simulink model "model_450"  (R2019b)
settings: Solver=VariableStepAuto  StartTime=0.0  StopTime=10  RelTol=3
libraries: powerlib x15, powerlib_meascontrol x3, eePwmGenerator x1
settings Model: Creator=Администратор  LastModifiedBy=Андрей
settings SFSimCC: CustomCodeUndefinedFunction=UseInterfaceOnly

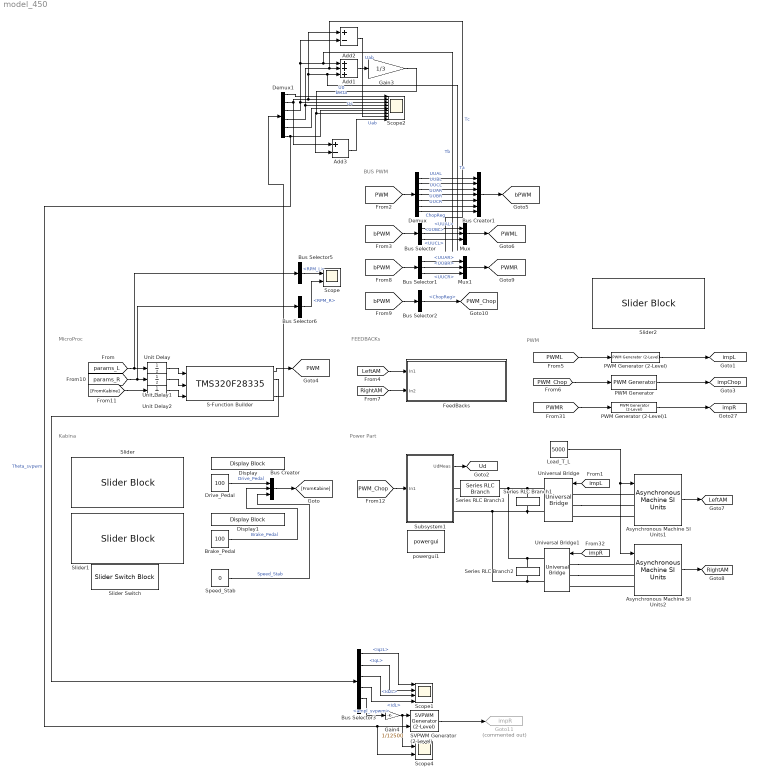
== system model_450 ==
  note: MiсroProc
  note: Kabina
  note: FEEDBACKs
  note: PWM
  note: Power Part
  note: BUS PWM
  Add1 : Sum  Inputs=+++
  Add2 : Sum  Inputs=+-
  Add3 : Sum  Inputs=+-
  Asynchronous Machine SI Units1 : powerlib/Machines/Asynchronous Machine SI Units  RotorType=Squirrel-cage  PresetModel=No  MechanicalLoad=Torque Tm  ShowDetailedParameters=on  ReferenceFrame=Rotor  Units=SI  MeasurementBus=off  NominalParameters=[800000 425 30]  Stator=[0.005 0.00015]  Rotor=[0.00483 0.00015]  Cage1=[ 0.022 0.226/377]  Cage2=[ 0.022 0.226/377]  Lm=0.0072  Mechanical=[100 0 3]  PolePairs=2  InitialConditions=[1 0 0 0 0 0 0 0]  SimulateSaturation=off  Saturation=[14.03593122, 27.81365428, 53.79336849, 72.68890987, 97.98006896, 148.6815601, 215.7428561, 302.9841135, 420.4778367 ; 230, 322, 414, 460, 506, 552, 598, 644, 690]  LoadFlowParameters=1492000  TsPowergui=0  TsBlock=-1  IterativeModel=Trapezoidal non iterative  IterativeDiscreteModel=Trapezoidal non iterative  Pmec=0
      settings: SourceProductName=Simscape Electrical
  Asynchronous Machine SI Units2 : powerlib/Machines/Asynchronous Machine SI Units  RotorType=Squirrel-cage  PresetModel=No  MechanicalLoad=Torque Tm  ShowDetailedParameters=on  ReferenceFrame=Rotor  Units=SI  MeasurementBus=off  NominalParameters=[800000 425 30]  Stator=[0.005 0.00015]  Rotor=[0.00483 0.00015]  Cage1=[ 0.022 0.226/377]  Cage2=[ 0.022 0.226/377]  Lm=0.0072  Mechanical=[100 0 3]  PolePairs=2  InitialConditions=[1 0 0 0 0 0 0 0]  SimulateSaturation=off  Saturation=[14.03593122, 27.81365428, 53.79336849, 72.68890987, 97.98006896, 148.6815601, 215.7428561, 302.9841135, 420.4778367 ; 230, 322, 414, 460, 506, 552, 598, 644, 690]  LoadFlowParameters=1492000  TsPowergui=0  TsBlock=-1  IterativeModel=Trapezoidal non iterative  IterativeDiscreteModel=Trapezoidal non iterative  Pmec=0
      settings: SourceProductName=Simscape Electrical
  Brake_Pedal : Constant  Value=100
  Bus Creator : BusCreator  Inputs=3
  Bus Creator1 : BusCreator  Inputs=7
  Bus Selector : BusSelector  OutputSignals=UUAL,UUBL,UUCL
  Bus Selector1 : BusSelector  OutputSignals=UUAR,UUBR,UUCR
  Bus Selector2 : BusSelector  OutputSignals=ChopReg
  Bus Selector3 : BusSelector  OutputSignals=IqzL,IqL,IdzL,IdL,ampl_svpwm,fThetaL
  Bus Selector5 : BusSelector  OutputSignals=RPM_L
  Bus Selector6 : BusSelector  OutputSignals=RPM_R
  Demux : Demux  Outputs=7
  Demux1 : Demux  Outputs=6
  Display : DisplayBlock  LabelPosition=Hide  Format=short
  Display1 : DisplayBlock  LabelPosition=Hide  Format=short
  Drive_Pedal : Constant  Value=100
  FeedBacks : Subsystem
  Gain3 : Gain  Gain=1/3
  Gain4 : Gain  Gain=1/12500
  Goto11 : Goto  Commented=on  GotoTag=impR  TagVisibility=global
  Load_T_L : Constant  Value=5000
  Mux : Mux  Inputs=3
  Mux1 : Mux  Inputs=3
  PWM Generator : eePwmGenerator/PWM Generator  CarrCount=Up  Tper=0.000666  Ts=1e-5
      settings: SourceProductName=Simscape Electrical
  PWM Generator (2-Level) : powerlib_meascontrol/Pulse & Signal Generators/PWM Generator (2-Level)  ModulatorType=Three-phase bridge (6 pulses)  ModulatorMode=Unsynchronized  Fc=1500  Pc=90  nF=27  MinMax="[ 0  25000 ]"  SamplingTechnique=Natural  ModulatingSignals=off  m=0.8  Freq=60  Phase=0  Ts=0  ShowCarrierOutport=off
  PWM Generator (2-Level)1 : powerlib_meascontrol/Pulse & Signal Generators/PWM Generator (2-Level)  ModulatorType=Three-phase bridge (6 pulses)  ModulatorMode=Unsynchronized  Fc=1500  Pc=90  nF=27  MinMax=[ 0 25000]  SamplingTechnique=Natural  ModulatingSignals=off  m=0.8  Freq=60  Phase=0  Ts=0  ShowCarrierOutport=off
  S-Function Builder : S-Function  InitFcn=try, set_param(gcb,'FunctionName','TMS320F28335'), end  FunctionName=TMS320F28335  SFunctionModules=TMS320F28335_wrapper RegL RegR func  SFunctionDeploymentMode=off  EnableBusSupport=off  mask(S-Function Builder){}
      mask help: Simulink:masks:SFunctionBuilder_MD
      mask init:
      | val = [[.9  0.75 0.75 1 1 .9 .9 1]',[1 1 0.75 0.75 .9 .9 1 .9]'];try , sys = get_param(gcb,'SfunBuilderFcnName');if isempty(sys), sys = get_param(gcb,'FunctionName'); end,catch, sys = get_param(gcb,'FunctionName'); end
      settings: CopyFcn=set_param(gcbh,'LinkStatus','none')  PreSaveFcn=try, set_param(gcb,'FunctionName','TMS320F28335'), end  OpenFcn=sfunctionwizard(gcbh)
      mask Display:
      | plot(val(:,1),val(:,2))
      | disp(sys)
      | port_label('input',1,'Lpars')
      | port_label('input',2,'Rpars')
      | port_label('input',3,'FromKabine')
      | port_label('output',1,'PWM')
      | port_label('output',2,'Out_L')
      | port_label('output',3,'Out_R')
      | port_label('output',4,'SVPWM')
  SVPWM Generator (2-Level) : powerlib_meascontrol/Pulse & Signal Generators/SVPWM Generator (2-Level)  InputType=Magnitude-Angle (rad)  SwitchingPattern=Pattern #1  Fc=1000  ParUref=[0.8 -30 50]  Ts=0
      settings: SourceProductName=Simscape Electrical  SourceProductBaseCode=PS
  Scope : Scope  NumInputPorts=2
  Scope1 : Scope  NumInputPorts=4
  Scope2 : Scope  NumInputPorts=9
  Scope4 : Scope  NumInputPorts=2
  Series RLC Branch1 : powerlib/Elements/Series RLC Branch  LConnTagsString=__new0  RConnTagsString=__new0  BranchType=C  Resistance=0.005  Inductance=1e-3  SetiL0=off  InitialCurrent=0  Capacitance=11e-3  Setx0=off  InitialVoltage=0  Measurements=None
      settings: SourceProductName=Simscape Electrical
  Series RLC Branch2 : powerlib/Elements/Series RLC Branch  LConnTagsString=__new0  RConnTagsString=__new0  BranchType=C  Resistance=0.005  Inductance=1e-3  SetiL0=off  InitialCurrent=0  Capacitance=11e-3  Setx0=off  InitialVoltage=0  Measurements=None
      settings: SourceProductName=Simscape Electrical
  Series RLC Branch3 : powerlib/Elements/Series RLC Branch  LConnTagsString=__new0  RConnTagsString=__new0  BranchType=R  Resistance=0.001  Inductance=1e-3  SetiL0=off  InitialCurrent=0  Capacitance=1e-6  Setx0=off  InitialVoltage=0  Measurements=None
      settings: SourceProductName=Simscape Electrical
  Slider : SliderBlock  TickInterval=10
  Slider Switch : SliderSwitchBlock
      settings: Values={{'Off', 'On'}, [0 1]}
  Slider1 : SliderBlock  TickInterval=10
  Slider2 : SliderBlock  ScaleMin=-5000  ScaleMax=5000
  Speed_Stab : Constant  Value=0
  Subsystem1 : Subsystem
  Unit Delay : UnitDelay  SampleTime=-1  HasFrameUpgradeWarning=on
  Unit Delay1 : UnitDelay  SampleTime=-1  HasFrameUpgradeWarning=on
  Unit Delay2 : UnitDelay  SampleTime=-1  HasFrameUpgradeWarning=on
  Universal Bridge : powerlib/Power Electronics/Universal Bridge  Arms=3  SnubberResistance=1e4  SnubberCapacitance=inf  Device=IGBT / Diodes  Ron=1e-3  Lon=0  ForwardVoltages="[  0  0  ]"  ForwardVoltage=0  GTOparameters=[ 10e-6 , 20e-6 ]  IGBTparameters=[ 0 , 0 ]  Measurements=None  Measurements_2=None  converterType=Rectifier
      settings: SourceProductName=Simscape Electrical
  Universal Bridge1 : powerlib/Power Electronics/Universal Bridge  Arms=3  SnubberResistance=1e4  SnubberCapacitance=inf  Device=IGBT / Diodes  Ron=1e-3  Lon=0  ForwardVoltages="[  0  0  ]"  ForwardVoltage=0  GTOparameters=[ 10e-6 , 20e-6 ]  IGBTparameters=[ 0 , 0 ]  Measurements=None  Measurements_2=None  converterType=Rectifier
      settings: SourceProductName=Simscape Electrical
  powergui1 : powerlib/powergui  Priority=1  SimulationMode=Discrete  SampleTime=2e-5  frequency=60  Iterations=50  frequencyindice=0  Pbase=100e6  ErrMax=1e-4  UnitsV=kV  UnitsW=MW  buscounter=0  FunctionMessages=off  echomessages=off  EnableUseOfTLC=off  CurrentSourceSwitches=off  DisableSnubberDevices=off  DisableRonSwitches=off  DisableVfSwitches=off  DisplayEquations=off  AutomaticDiscreteSolvers=off  SolverType=Backward Euler  Interpol=off  ExternalGateDelay=off  methode=off  Ts=0  x0status=blocks  SPID=off  SwTol=0  HookPort=off  NonlinearTolerance=0  nMaxIteration=15  ContinueOnMaxIteration=off  RestoreLinks=warning  ResistiveCurrentMeasurement=off  Frange=[0:2:500]  Ylog=off  Xlog=on  ShowGrid=off  save=off  variable=ZData  structure=0  ZoomFFT=off  StartTime=0.0  cycles=1  DisplayStyle=1  fundamental=60  FreqAxis=off  MaxFrequency=1000  frequencyindicesteady=1  RmsSteady=1  display=off
      settings: SourceProductName=Simscape Electrical
  tag scope: LeftAM=global, PWM=global, PWML=global, PWMR=global, PWM_Chop=global, RightAM=global, Ud=global, bPWM=global, impChop=global, impL=global, impR=global
  wires:
  Subsystem1/1(UdMeas) -> [Ud]
  [RightAM] -> FeedBacks/2(In2)
  [PWML] -> PWM Generator (2-Level)/1
  PWM Generator/1 -> [impChop]
  Bus Selector/2 -> Mux/2  "<UUBL>"
  Mux/1 -> [PWML]
  [PWM_Chop] -> Subsystem1/1(In1)
  Demux/6 -> Bus Creator1/6  "UUCR"
  [impR] -> Universal Bridge1/1
  Bus Selector1/1 -> Mux1/1  "<UUAR>"
  Bus Creator/1 -> [FromKabine]
  S-Function Builder/1 -> [PWM]
  Demux/3 -> Bus Creator1/3  "UUCL"
  Bus Selector2/1 -> [PWM_Chop]  "<ChopReg>"
  Bus Selector/3 -> Mux/3  "<UUCL>"
  Asynchronous Machine SI Units2/1 -> [RightAM]
  Demux/7 -> Bus Creator1/7  "ChopReg"
  [PWM_Chop] -> PWM Generator/1
  Bus Selector1/3 -> Mux1/3  "<UUCR>"
  Mux1/1 -> [PWMR]
  Demux/4 -> Bus Creator1/4  "UUAR"
  Bus Selector1/2 -> Mux1/2  "<UUBR>"
  Speed_Stab/1 -> Bus Creator/3  "Speed_Stab"
  [bPWM] -> Bus Selector/1
  [params_R] -> Bus Selector6/1, Unit Delay1/1
  [PWM] -> Demux/1
  Bus Selector/1 -> Mux/1  "<UUAL>"
  Asynchronous Machine SI Units1/1 -> [LeftAM]
  Demux/1 -> Bus Creator1/1  "UUAL"
  [FromKabine] -> Unit Delay2/1
  [LeftAM] -> FeedBacks/1(In1)
  [impL] -> Universal Bridge/1
  Unit Delay/1 -> S-Function Builder/1
  [PWMR] -> PWM Generator (2-Level)1/1
  Unit Delay2/1 -> S-Function Builder/3
  Brake_Pedal/1 -> Bus Creator/2  "Brake_Pedal"
  Drive_Pedal/1 -> Bus Creator/1  "Drive_Pedal"
  Demux/5 -> Bus Creator1/5  "UUBR"
  Bus Creator1/1 -> [bPWM]
  [params_L] -> Bus Selector5/1, Unit Delay/1
  [bPWM] -> Bus Selector1/1
  PWM Generator (2-Level)1/1 -> [impR]
  Demux/2 -> Bus Creator1/2  "UUBL"
  [bPWM] -> Bus Selector2/1
  PWM Generator (2-Level)/1 -> [impL]
  Unit Delay1/1 -> S-Function Builder/2
  SVPWM Generator (2-Level)/1 -> Goto11/1
  Bus Selector3/2 -> Scope1/2  "<IqL>"
  Bus Selector3/4 -> Scope1/4  "<IdL>"
  Bus Selector3/3 -> Scope1/3  "<IdzL>"
  Bus Selector3/1 -> Scope1/1  "<IqzL>"
  Bus Selector3/5 -> Gain4/1  "<ampl_svpwm>"
  Gain4/1 -> Scope4/1, SVPWM Generator (2-Level)/1
  Demux1/2 -> Add3/1, Add2/1, Add1/3, Scope2/2  "Ta"
  Add1/1 -> Gain3/1
  Demux1/5 -> Scope2/5  "Us"
  Gain3/1 -> Add3/2, Scope2/7  "U0"
  Add2/1 -> Scope2/8  "Uab"
  Add3/1 -> Scope2/9  "Uab"
  Demux1/4 -> Add1/2, Scope2/4  "Tc"
  Demux1/1 -> Scope2/1  "betta"
  Demux1/3 -> Add2/2, Add1/1, Scope2/3  "Tb"
  Demux1/6 -> Scope4/2, SVPWM Generator (2-Level)/2, Scope2/6  "Theta_svpwm"
  Load_T_L/1 -> Asynchronous Machine SI Units1/1, Asynchronous Machine SI Units2/1
  Bus Selector6/1 -> Scope/2  "<RPM_R>"
  Bus Selector5/1 -> Scope/1  "<RPM_L>"
  S-Function Builder/4 -> Demux1/1
  S-Function Builder/2 -> Bus Selector3/1
  connections:
  Series RLC Branch3/LConn1 -- Universal Bridge1/RConn1 -- Series RLC Branch2/LConn1 -- Universal Bridge/RConn1 -- Series RLC Branch1/LConn1
  Series RLC Branch1/RConn1 -- Subsystem1/RConn2 -- Universal Bridge1/RConn2 -- Series RLC Branch2/RConn1 -- Universal Bridge/RConn2
  Asynchronous Machine SI Units1/LConn1 -- Universal Bridge/LConn1
  Universal Bridge1/LConn1 -- Asynchronous Machine SI Units2/LConn1
  Universal Bridge/LConn2 -- Asynchronous Machine SI Units1/LConn2
  Asynchronous Machine SI Units1/LConn3 -- Universal Bridge/LConn3
  Universal Bridge1/LConn2 -- Asynchronous Machine SI Units2/LConn2
  Series RLC Branch3/RConn1 -- Subsystem1/RConn1
  Asynchronous Machine SI Units2/LConn3 -- Universal Bridge1/LConn3

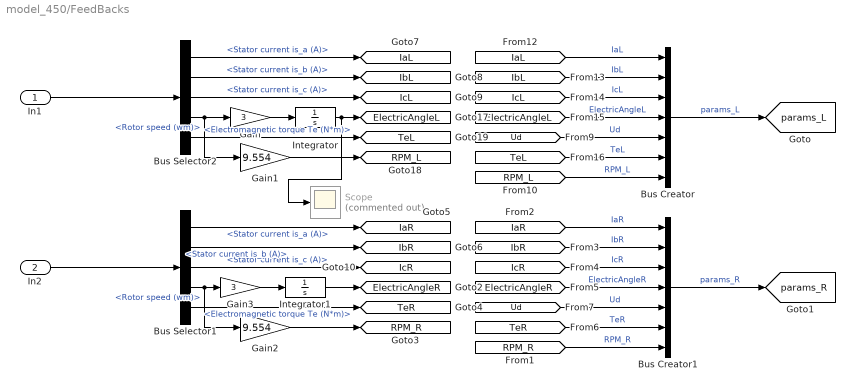
== system model_450/FeedBacks ==
  In1 : Inport
  In2 : Inport  Port=2
  Bus Creator : BusCreator  Inputs=7
  Bus Creator1 : BusCreator  Inputs=7
  Bus Selector1 : BusSelector  OutputSignals=Stator measurements.Stator current is_a (A),Stator measurements.Stator current is_b (A),Stator measurements.Stator current is_c (A),Mechanical.Rotor speed (wm),Mechanical.Electromagnetic torque Te (N*m)
  Bus Selector2 : BusSelector  OutputSignals=Stator measurements.Stator current is_a (A),Stator measurements.Stator current is_b (A),Stator measurements.Stator current is_c (A),Mechanical.Rotor speed (wm),Mechanical.Electromagnetic torque Te (N*m)
  Gain : Gain  Gain=3
  Gain1 : Gain  Gain=9.554
  Gain2 : Gain  Gain=9.554
  Gain3 : Gain  Gain=3
  Integrator : Integrator  WrapState=on  WrappedStateUpperValue=2*pi  WrappedStateLowerValue=0
  Integrator1 : Integrator  WrapState=on  WrappedStateUpperValue=2*pi  WrappedStateLowerValue=0
  Scope : Scope  Commented=on
  tag scope: ElectricAngleL=global, ElectricAngleR=global, IaL=global, IaR=global, IbL=global, IbR=global, IcL=global, IcR=global, RPM_L=global, RPM_R=global, TeL=global, TeR=global, params_L=global, params_R=global
  wires:
  [TeL] -> Bus Creator/6  "TeL"
  Bus Selector2/3 -> [IcL]  "<Stator current is_c (A)>"
  In1/1 -> Bus Selector2/1
  [IaL] -> Bus Creator/1  "IaL"
  Bus Selector2/4 -> Gain1/1, Gain/1  "<Rotor speed (wm)>"
  Bus Selector2/2 -> [IbL]  "<Stator current is_b (A)>"
  [IbL] -> Bus Creator/2  "IbL"
  Bus Selector2/1 -> [IaL]  "<Stator current is_a (A)>"
  [ElectricAngleL] -> Bus Creator/4  "ElectricAngleL"
  Bus Selector2/5 -> [TeL]  "<Electromagnetic torque Te (N*m)>"
  Gain1/1 -> [RPM_L]
  [RPM_L] -> Bus Creator/7  "RPM_L"
  [Ud] -> Bus Creator/5  "Ud"
  [IcL] -> Bus Creator/3  "IcL"
  Bus Creator/1 -> [params_L]  "params_L"
  [IcR] -> Bus Creator1/3  "IcR"
  [IaR] -> Bus Creator1/1  "IaR"
  [Ud] -> Bus Creator1/5  "Ud"
  Bus Selector1/4 -> Gain3/1, Gain2/1  "<Rotor speed (wm)>"
  Bus Creator1/1 -> [params_R]  "params_R"
  [ElectricAngleR] -> Bus Creator1/4  "ElectricAngleR"
  [IbR] -> Bus Creator1/2  "IbR"
  [TeR] -> Bus Creator1/6  "TeR"
  Gain2/1 -> [RPM_R]
  [RPM_R] -> Bus Creator1/7  "RPM_R"
  Bus Selector1/1 -> [IaR]  "<Stator current is_a (A)>"
  Bus Selector1/5 -> [TeR]  "<Electromagnetic torque Te (N*m)>"
  Bus Selector1/3 -> [IcR]  "<Stator current is_c (A)>"
  Bus Selector1/2 -> [IbR]  "<Stator current is_b (A)>"
  In2/1 -> Bus Selector1/1
  Integrator/1 -> Scope/1, [ElectricAngleL]
  Gain/1 -> Integrator/1
  Integrator1/1 -> [ElectricAngleR]
  Gain3/1 -> Integrator1/1

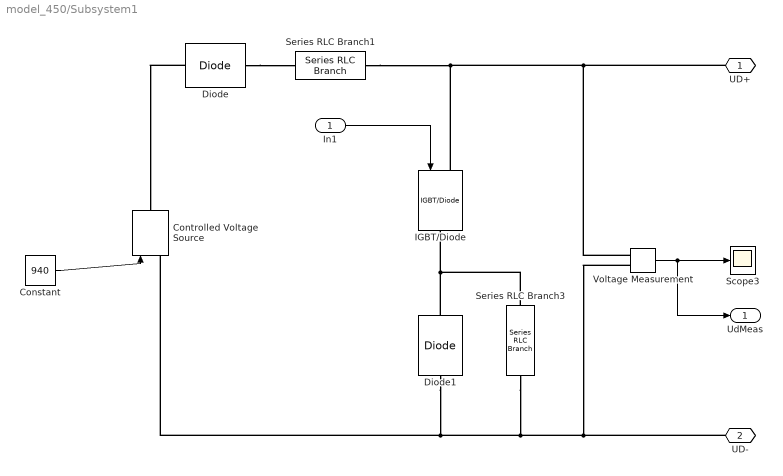
== system model_450/Subsystem1 ==
  In1 : Inport
  Constant : Constant  Value=940
  Controlled Voltage Source : powerlib/Electrical Sources/Controlled Voltage Source  Initialize=on  Source_Type=AC  Amplitude=0  Phase=0  Frequency=0  Measurements=None
      settings: SourceProductName=Simscape Electrical
  Diode : powerlib/Power Electronics/Diode  Ron=0.001  Lon=0  Vf=0.8  IC=0  UseSnubber=0  Rs=500  Cs=250e-9  Measurements=off
      settings: SourceProductName=Simscape Electrical
  Diode1 : powerlib/Power Electronics/Diode  Ron=0.001  Lon=0  Vf=0.8  IC=0  UseSnubber=0  Rs=500  Cs=250e-9  Measurements=off
      settings: SourceProductName=Simscape Electrical
  IGBT/Diode : powerlib/Power Electronics/IGBT//Diode  Ron=1e-3  Rs=1e5  Cs=inf  Measurements=off
      settings: SourceProductName=Simscape Electrical
  Scope3 : Scope
  Series RLC Branch1 : powerlib/Elements/Series RLC Branch  LConnTagsString=__new0  RConnTagsString=__new0  BranchType=R  Resistance=0.001  Inductance=1e-4  SetiL0=off  InitialCurrent=0  Capacitance=1e-6  Setx0=off  InitialVoltage=0  Measurements=None
      settings: SourceProductName=Simscape Electrical
  Series RLC Branch3 : powerlib/Elements/Series RLC Branch  LConnTagsString=__new0  RConnTagsString=__new0  BranchType=R  Resistance=0.35  Inductance=1e-3  SetiL0=off  InitialCurrent=0  Capacitance=1e-6  Setx0=off  InitialVoltage=0  Measurements=None
      settings: SourceProductName=Simscape Electrical
  Voltage Measurement : powerlib/Measurements/Voltage Measurement  PhasorSimulation=off  OutputType=Complex  PSBequivalent=0
      settings: SourceProductName=Simscape Electrical
  UD+ : PMIOPort  Side=Right
  "UD- " : PMIOPort  Port=2  Side=Right
  UdMeas : Outport  VectorParamsAs1DForOutWhenUnconnected=off
  wires:
  Voltage Measurement/1 -> UdMeas/1, Scope3/1
  In1/1 -> IGBT/Diode/1
  Constant/1 -> Controlled Voltage Source/1
  connections:
  Voltage Measurement/LConn2 -- "UD- "/RConn1 -- Series RLC Branch3/RConn1 -- Controlled Voltage Source/LConn1 -- Diode1/LConn1
  Voltage Measurement/LConn1 -- UD+/RConn1 -- IGBT/Diode/LConn1 -- Series RLC Branch1/LConn1
  Diode1/RConn1 -- Series RLC Branch3/LConn1 -- IGBT/Diode/RConn1
  Diode/LConn1 -- Controlled Voltage Source/RConn1
  Diode/RConn1 -- Series RLC Branch1/RConn1
